simulink model "BlackBox"  (Simulink 8.8)
settings: Solver=ode45  StartTime=0.0  StopTime=100.0  RelTol=1e-3  EnableMultiTasking=on
undefined symbols (not defined in the file): Ts
settings Model: Creator=roadgont  LastModifiedBy=mariv
settings DataIOCC: SignalLoggingSaveFormat=Dataset
settings DebuggingCC: SolverPrmCheckMsg=warning  FcnCallInpInsideContextMsg=error
settings HardwareCC: TargetBitPerPointer=64  TargetBitPerSizeT=64  TargetBitPerPtrDiffT=64  TargetLongLongMode=on  TargetIntDivRoundTo=Zero  TargetEndianess=LittleEndian  TargetWordSize=64  TargetHWDeviceType=MATLAB Host  ProdEqTarget=off
settings RTWCC: SystemTargetFile=rtwsfcn.tlc  PackageGeneratedCodeAndArtifacts=on  PackageName=CajaNegra  TemplateMakefile=rtwsfcn_default_tmf  Description=S-Function Target  TargetLang=C++
settings STFCustomTargetCC: ModelReferenceCompliant=off  CompOptLevelCompliant=on  GeneratePreprocessorConditionals=Disable all  MATLABClassNameForMDSCustomization=Simulink.SoftwareTarget.TargetSpecificTriggerConfigurationBase  SystemTargetFile=rtwsfcn.tlc
settings CustomProperty: Value=on
settings ConfigComp: CovSFcnEnable=off

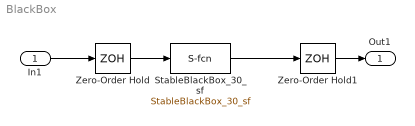
== system BlackBox ==
  In1 : Inport
  StableBlackBox_30_sf : S-Function  FunctionName=StableBlackBox_30_sf  SFunctionDeploymentMode=off  EnableBusSupport=off
  Zero-Order Hold : ZeroOrderHold  SampleTime=Ts
  Zero-Order Hold1 : ZeroOrderHold  SampleTime=Ts
  Out1 : Outport
  wires:
  Zero-Order Hold1/1 -> Out1/1
  In1/1 -> Zero-Order Hold/1
  Zero-Order Hold/1 -> StableBlackBox_30_sf/1
  StableBlackBox_30_sf/1 -> Zero-Order Hold1/1
